simulink library "LegIK"  (R2014b)
settings: Solver=ode45  StartTime=0.0  StopTime=10.0  RelTol=1e-3
settings Model: Creator=Sebastian  LastModifiedBy=Sebastian

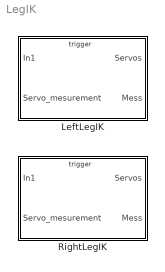
== system LegIK ==
  LeftLegIK : Subsystem  TreatAsAtomicUnit=on  RTWFcnName=LeftLegIK  mask{ID1=0, ID2=0, ID3=0}
      mask prompts: ID1 "Id servo 1"; ID2 "Id servo 2"; ID3 "Id servo 3"
      settings: RTWFcnNameOpts=User specified
  RightLegIK : Subsystem  TreatAsAtomicUnit=on  RTWFcnName=RightLegIK  mask{ID1=0, ID2=0, ID3=0}
      mask prompts: ID1 "Id servo 1"; ID2 "Id servo 2"; ID3 "Id servo 3"
      settings: RTWFcnNameOpts=User specified

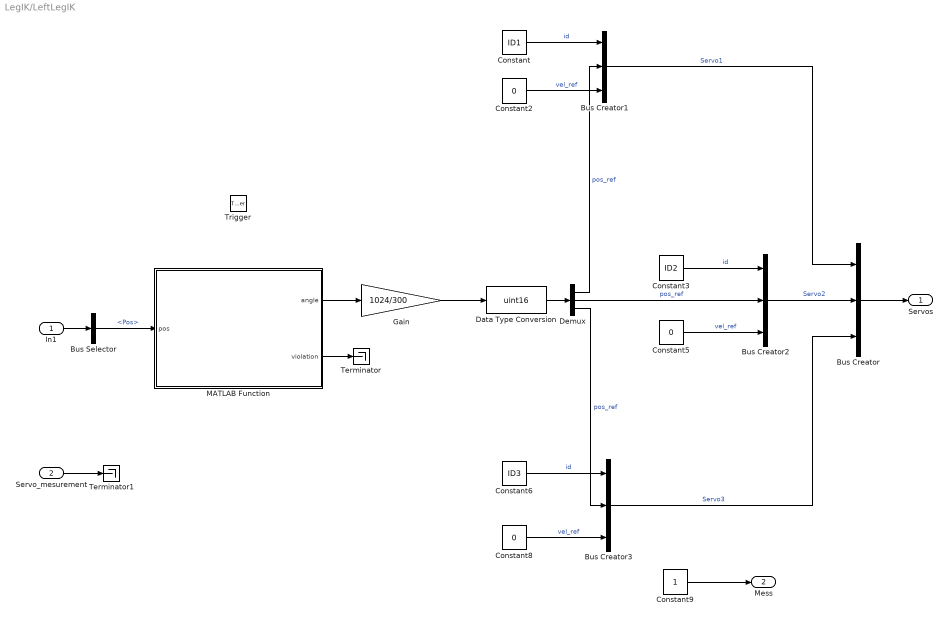
== system LegIK/LeftLegIK ==
  In1 : Inport  OutDataTypeStr=Bus: Leg_data
  Servo_mesurement : Inport  Port=2  OutDataTypeStr=Bus: Leg_mes
  Trigger : TriggerPort  PortDimensions=1
  Bus Creator : BusCreator  Inputs=3  OutDataTypeStr=Bus: Leg_ref  NonVirtualBus=on
      settings: InheritFromInputs=off
  Bus Creator1 : BusCreator  Inputs=3  OutDataTypeStr=Bus: Servo  NonVirtualBus=on
      settings: InheritFromInputs=off
  Bus Creator2 : BusCreator  Inputs=3  OutDataTypeStr=Bus: Servo  NonVirtualBus=on
      settings: InheritFromInputs=off
  Bus Creator3 : BusCreator  Inputs=3  OutDataTypeStr=Bus: Servo  NonVirtualBus=on
      settings: InheritFromInputs=off
  Bus Selector : BusSelector  OutputSignals=Pos
  Constant : Constant  Value=ID1  OutDataTypeStr=uint8  SampleTime=-1
  Constant2 : Constant  Value=0  OutDataTypeStr=uint16  SampleTime=-1
  Constant3 : Constant  Value=ID2  OutDataTypeStr=uint8  SampleTime=-1
  Constant5 : Constant  Value=0  OutDataTypeStr=uint16  SampleTime=-1
  Constant6 : Constant  Value=ID3  OutDataTypeStr=uint8  SampleTime=-1
  Constant8 : Constant  Value=0  OutDataTypeStr=uint16  SampleTime=-1
  Constant9 : Constant  OutDataTypeStr=uint16  SampleTime=-1
  Data Type Conversion : DataTypeConversion  OutDataTypeStr=uint16
  Demux : Demux  Outputs=3
  Gain : Gain  Gain=1024/300
  MATLAB Function : MATLAB Function  TreatAsAtomicUnit=on
  Terminator : Terminator
  Terminator1 : Terminator
  Servos : Outport  OutDataTypeStr=Bus: Leg_ref  PortDimensions=3
  Mess : Outport  Port=2
  wires:
  Bus Creator/1 -> Servos/1
  Bus Creator1/1 -> Bus Creator/1  "Servo1"
  Bus Creator2/1 -> Bus Creator/2  "Servo2"
  Constant/1 -> Bus Creator1/1  "id"
  Demux/1 -> Bus Creator1/2  "pos_ref"
  Bus Creator3/1 -> Bus Creator/3  "Servo3"
  Constant3/1 -> Bus Creator2/1  "id"
  Constant6/1 -> Bus Creator3/1  "id"
  Constant9/1 -> Mess/1
  Servo_mesurement/1 -> Terminator1/1
  Demux/3 -> Bus Creator3/2  "pos_ref"
  Demux/2 -> Bus Creator2/2  "pos_ref"
  Data Type Conversion/1 -> Demux/1
  In1/1 -> Bus Selector/1
  Gain/1 -> Data Type Conversion/1
  Constant2/1 -> Bus Creator1/3  "vel_ref"
  Constant5/1 -> Bus Creator2/3  "vel_ref"
  Constant8/1 -> Bus Creator3/3  "vel_ref"
  MATLAB Function/1(angle) -> Gain/1
  Bus Selector/1 -> MATLAB Function/1(pos)  "<Pos>"
  MATLAB Function/2(violation) -> Terminator/1

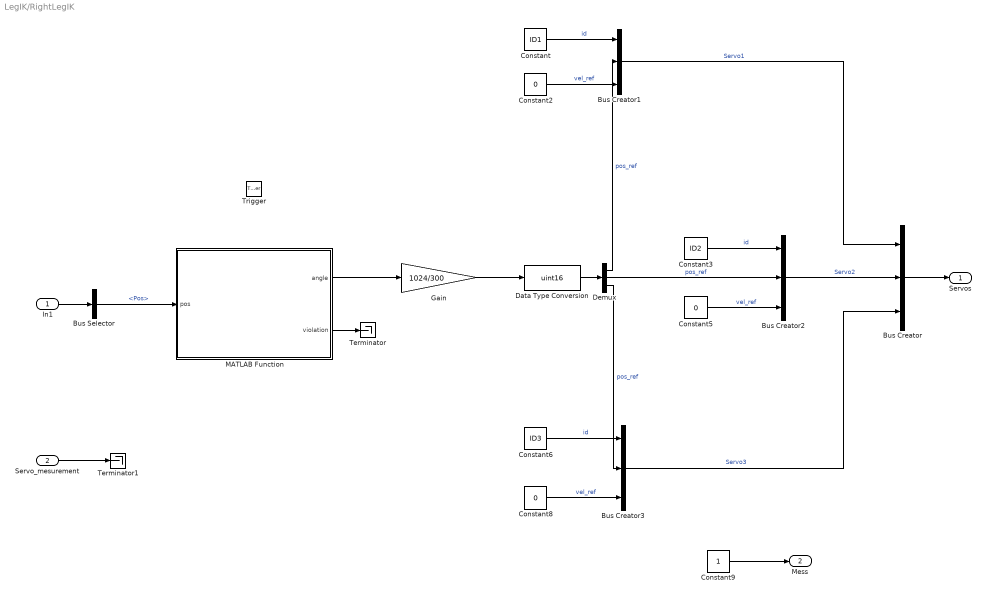
== system LegIK/RightLegIK ==
  In1 : Inport  OutDataTypeStr=Bus: Leg_data
  Servo_mesurement : Inport  Port=2  OutDataTypeStr=Bus: Leg_mes
  Trigger : TriggerPort  PortDimensions=1
  Bus Creator : BusCreator  Inputs=3  OutDataTypeStr=Bus: Leg_ref  NonVirtualBus=on
      settings: InheritFromInputs=off
  Bus Creator1 : BusCreator  Inputs=3  OutDataTypeStr=Bus: Servo  NonVirtualBus=on
      settings: InheritFromInputs=off
  Bus Creator2 : BusCreator  Inputs=3  OutDataTypeStr=Bus: Servo  NonVirtualBus=on
      settings: InheritFromInputs=off
  Bus Creator3 : BusCreator  Inputs=3  OutDataTypeStr=Bus: Servo  NonVirtualBus=on
      settings: InheritFromInputs=off
  Bus Selector : BusSelector  OutputSignals=Pos
  Constant : Constant  Value=ID1  OutDataTypeStr=uint8  SampleTime=-1
  Constant2 : Constant  Value=0  OutDataTypeStr=uint16  SampleTime=-1
  Constant3 : Constant  Value=ID2  OutDataTypeStr=uint8  SampleTime=-1
  Constant5 : Constant  Value=0  OutDataTypeStr=uint16  SampleTime=-1
  Constant6 : Constant  Value=ID3  OutDataTypeStr=uint8  SampleTime=-1
  Constant8 : Constant  Value=0  OutDataTypeStr=uint16  SampleTime=-1
  Constant9 : Constant  OutDataTypeStr=uint16
  Data Type Conversion : DataTypeConversion  OutDataTypeStr=uint16
  Demux : Demux  Outputs=3
  Gain : Gain  Gain=1024/300
  MATLAB Function : MATLAB Function  TreatAsAtomicUnit=on
  Terminator : Terminator
  Terminator1 : Terminator
  Servos : Outport  OutDataTypeStr=Bus: Leg_ref  PortDimensions=3
  Mess : Outport  Port=2
  wires:
  In1/1 -> Bus Selector/1
  Servo_mesurement/1 -> Terminator1/1
  Constant9/1 -> Mess/1
  Gain/1 -> Data Type Conversion/1
  Bus Creator/1 -> Servos/1
  Bus Creator1/1 -> Bus Creator/1  "Servo1"
  Bus Creator2/1 -> Bus Creator/2  "Servo2"
  Constant/1 -> Bus Creator1/1  "id"
  Demux/1 -> Bus Creator1/2  "pos_ref"
  Bus Creator3/1 -> Bus Creator/3  "Servo3"
  Constant3/1 -> Bus Creator2/1  "id"
  Constant6/1 -> Bus Creator3/1  "id"
  Demux/3 -> Bus Creator3/2  "pos_ref"
  Demux/2 -> Bus Creator2/2  "pos_ref"
  Data Type Conversion/1 -> Demux/1
  Constant2/1 -> Bus Creator1/3  "vel_ref"
  Constant5/1 -> Bus Creator2/3  "vel_ref"
  Constant8/1 -> Bus Creator3/3  "vel_ref"
  MATLAB Function/1(angle) -> Gain/1
  Bus Selector/1 -> MATLAB Function/1(pos)  "<Pos>"
  MATLAB Function/2(violation) -> Terminator/1

== matlab function LegIK/LeftLegIK/MATLAB Function ==
  data: pos input; angle output; violation output
function [angle, violation] = fcn(pos)
%Calibration values to measure offset for each angle
%x=0 y=209.4 z=93.8 
angle=zeros(1,3);

x=pos(1);
y=pos(2);
z=pos(3);

Coxa=53;%tidigare 52
Femur=66;%From CAD model 66.3456 mm
Tibia=133;%From CAD model 133.1793 mm


trueX=sqrt(x^2+y^2)-Coxa;

z=z+17.6;%Distance from bottom plate to coxa center
L=sqrt(trueX^2+z^2);
L2=L^2;

%Cox angle
angle(1)=atan2d(x,y);

%Femur angle
alpha1=atan2d(z,trueX);
alpha2=acosd((Femur^2+L2-Tibia^2)/(2*Femur*L));
angle(2)=alpha2-alpha1+13.6867;


%Tibia angle
beta=(Tibia^2+Femur^2-L2)/(2*Tibia*Femur);
angle(3)=acosd(beta)-147.6177;

angle=150-angle;

[angle, violation] = testConstraints(angle);

function [angle, violation] = testConstraints(angle)
persistent max;
persistent min;
if isempty(max)
    max = [810 810 840].*0.29;
end
if isempty(min)
    min = [220 210 320].*0.29;
end
violation = 0;

for i = 1:3
    if angle(i) < min(i)
        angle(i) = min(i);
        violation = i;
    end
    if angle(i) > max(i)
        angle(i) = max(i);
        violation = i;
    end
end

== matlab function LegIK/RightLegIK/MATLAB Function ==
  data: pos input; angle output; violation output
function [angle, violation] = fcn(pos)
%Calebration values (mm)
%x=0 y=209.4 z=93.8 

angle=zeros(1,3);

x=pos(1);
y=pos(2);
z=pos(3);

Coxa=53;
Femur=66;%From CAD model  66.3456 mm
Tibia=133;%From CAD model  133.1793 mm


trueX=sqrt(x^2+y^2)-Coxa;
z=z+17.6;%Distance from bottom plate to coxa center
L=sqrt(trueX^2+z^2);
L2=L^2;

%Cox angle
angle(1)=-atan2d(x,y);


%Femur angle
alpha1=atan2d(z,trueX);
alpha2=acosd((Femur^2+L2-Tibia^2)/(2*Femur*L));
angle(2)=alpha2-alpha1+13.6867;


%Tibia angle
beta=(Tibia^2+Femur^2-L2)/(2*Tibia*Femur);
angle(3)=acosd(beta)-147.6177;

angle=150+angle;

[angle, violation] = testConstraints(angle);


function [angle, violation] = testConstraints(angle)
persistent max;
persistent min;
if isempty(max)
    max = [810 810 660].*0.29;
end
if isempty(min)
    min = [220 210 170].*0.29;
end
violation = 0;

for i = 1:3
    if angle(i) < min(i)
        angle(i) = min(i);
        violation = i;
    end
    if angle(i) > max(i)
        angle(i) = max(i);
        violation = i;
    end
end
